simulink model "rhszero"  (R2014b)
settings: Solver=ode45  StartTime=0.0  StopTime=10.0  RelTol=1e-3
settings Model: Creator=kjartan  LastModifiedBy=kjartan

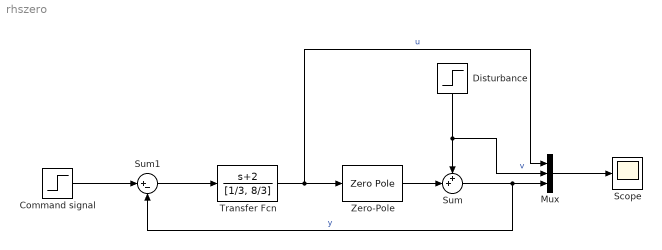
== system rhszero ==
  Command signal : Step  Time=0  SampleTime=0
  Disturbance : Step  Time=5  After=-1  SampleTime=0
  Mux : Mux  Inputs=3
  Scope : Scope
      settings: ShowLegends=on
  Sum : Sum  Inputs=++|
  Sum1 : Sum  Inputs=|+-
  Transfer Fcn : TransferFcn  Numerator=[1, 2]  Denominator=[1/3, 8/3]
  Zero-Pole : ZeroPole  Zeros=[2]  Poles=[0, -2]  Gain=[-1]
  wires:
  Sum/1 -> Sum1/2, Mux/3  "y"
  Zero-Pole/1 -> Sum/2
  Transfer Fcn/1 -> Mux/1, Zero-Pole/1  "u"
  Sum1/1 -> Transfer Fcn/1
  Mux/1 -> Scope/1
  Command signal/1 -> Sum1/1
  Disturbance/1 -> Mux/2, Sum/1  "v"
